simulink model "controller_v9"  (R2022b)
settings: Solver=ode4  StartTime=0.0  StopTime=5  FixedStep=0.00001  RelTol=1e-3
values from neighbouring files (symbols this model uses):
  m = 6    [coordinator_v2.m]
  N = 10    [coordinator_v2.m]
undefined symbols (not defined in the file or in its folder): PD_result, sd, X, Y, Z
libraries: sm_lib x191, nesl_utility x71
(part 2 of 5)

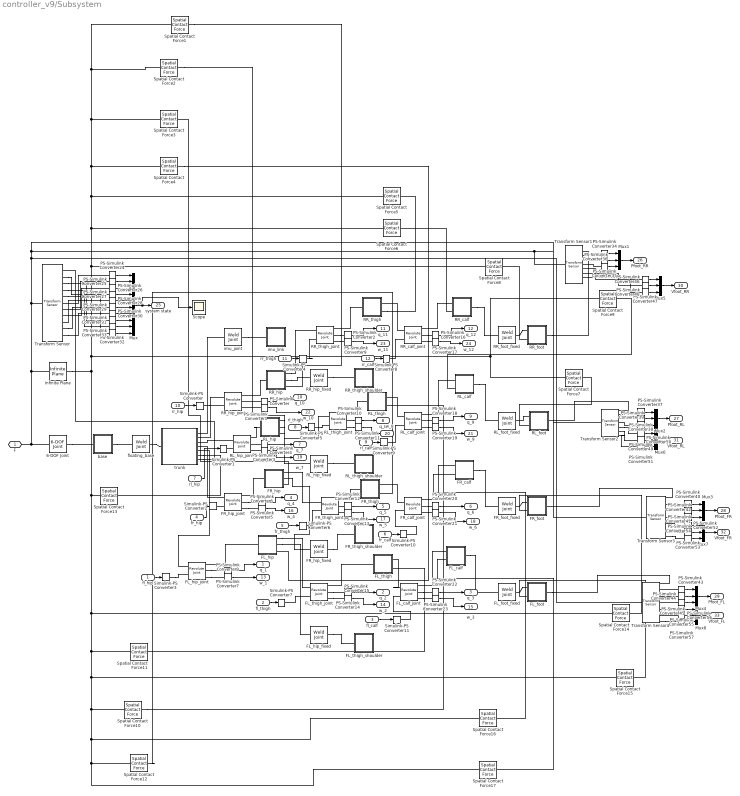
== system controller_v9/Subsystem ==
  fl_hip : Inport
  fl_thigh : Inport  Port=2
  fl_calf : Inport  Port=3
  fr_hip : Inport  Port=4
  fr_thigh : Inport  Port=5
  fr_calf : Inport  Port=6
  rl_hip : Inport  Port=7
  rl_thigh : Inport  Port=8
  rl_calf : Inport  Port=9
  rr_hip : Inport  Port=10
  rr_thigh : Inport  Port=11
  rr_calf : Inport  Port=12
  6-DOF Joint : sm_lib/Joints/6-DOF Joint  JointMode=Normal  SenseConstraintForce=off  SenseConstraintForceX=off  SenseConstraintForceY=off  SenseConstraintForceZ=off  SenseConstraintTorque=off  SenseConstraintTorqueX=off  SenseConstraintTorqueY=off  SenseConstraintTorqueZ=off  SenseTotalForce=off  SenseTotalForceX=off  SenseTotalForceY=off  SenseTotalForceZ=off  SenseTotalTorque=off  SenseTotalTorqueX=off  SenseTotalTorqueY=off  SenseTotalTorqueZ=off  CompositeWrenchDir=FollowerOnBase  CompositeWrenchFrame=BaseFrame  PxEquilibriumPosition=0  PxEquilibriumPositionUnits=m  PxSpringStiffness=0  PxSpringStiffnessUnits=N/m  PxDampingCoefficient=0  PxDampingCoefficientUnits=N/(m/s)  PxTorqueActuationMode=NoTorque  PxMotionActuationMode=ComputedMotion  PxSensePosition=off  PxSenseVelocity=off  PxSenseAcceleration=off  PxSenseTorqueForce=off  PxSenseLowerLimitTorqueForce=off  PxSenseUpperLimitTorqueForce=off  PxLowerLimitSpecify=off  PxLowerLimitBound=-1  PxLowerLimitBoundUnits=m  PxLowerLimitStiffness=1e6  PxLowerLimitStiffnessUnits=N/m  PxLowerLimitDamping=1e3  PxLowerLimitDampingUnits=N/(m/s)  PxLowerLimitTransitionRegionWidth=1e-4  PxLowerLimitTransitionRegionWidthUnits=m  PxUpperLimitSpecify=off  PxUpperLimitBound=1  PxUpperLimitBoundUnits=m  PxUpperLimitStiffness=1e6  PxUpperLimitStiffnessUnits=N/m  PxUpperLimitDamping=1e3  PxUpperLimitDampingUnits=N/(m/s)  PxUpperLimitTransitionRegionWidth=1e-4  PxUpperLimitTransitionRegionWidthUnits=m  PxPositionTargetSpecify=off  PxPositionTargetPriority=High  PxPositionTargetValue=0  PxPositionTargetValueUnits=m  PxVelocityTargetSpecify=off  PxVelocityTargetPriority=High  PxVelocityTargetValue=0  PxVelocityTargetValueUnits=m/s  PyEquilibriumPosition=0  PyEquilibriumPositionUnits=m  PySpringStiffness=0  PySpringStiffnessUnits=N/m  PyDampingCoefficient=0  PyDampingCoefficientUnits=N/(m/s)  PyTorqueActuationMode=NoTorque  PyMotionActuationMode=ComputedMotion  PySensePosition=off  PySenseVelocity=off  PySenseAcceleration=off  PySenseTorqueForce=off  PySenseLowerLimitTorqueForce=off  PySenseUpperLimitTorqueForce=off  PyLowerLimitSpecify=off  PyLowerLimitBound=-1  PyLowerLimitBoundUnits=m  PyLowerLimitStiffness=1e6  PyLowerLimitStiffnessUnits=N/m  PyLowerLimitDamping=1e3  PyLowerLimitDampingUnits=N/(m/s)  PyLowerLimitTransitionRegionWidth=1e-4  PyLowerLimitTransitionRegionWidthUnits=m  PyUpperLimitSpecify=off  PyUpperLimitBound=1  PyUpperLimitBoundUnits=m  PyUpperLimitStiffness=1e6  PyUpperLimitStiffnessUnits=N/m  PyUpperLimitDamping=1e3  PyUpperLimitDampingUnits=N/(m/s)  PyUpperLimitTransitionRegionWidth=1e-4  PyUpperLimitTransitionRegionWidthUnits=m  PyPositionTargetSpecify=off  PyPositionTargetPriority=High  PyPositionTargetValue=0  PyPositionTargetValueUnits=m  PyVelocityTargetSpecify=off  PyVelocityTargetPriority=High  PyVelocityTargetValue=0  PyVelocityTargetValueUnits=m/s  PzEquilibriumPosition=0  PzEquilibriumPositionUnits=m  PzSpringStiffness=0  PzSpringStiffnessUnits=N/m  PzDampingCoefficient=0  PzDampingCoefficientUnits=N/(m/s)  PzTorqueActuationMode=NoTorque  PzMotionActuationMode=ComputedMotion  PzSensePosition=off  PzSenseVelocity=off  PzSenseAcceleration=off  PzSenseTorqueForce=off  PzSenseLowerLimitTorqueForce=off  PzSenseUpperLimitTorqueForce=off  PzLowerLimitSpecify=off  PzLowerLimitBound=-1  PzLowerLimitBoundUnits=m  PzLowerLimitStiffness=1e6  PzLowerLimitStiffnessUnits=N/m  PzLowerLimitDamping=1e3  PzLowerLimitDampingUnits=N/(m/s)  PzLowerLimitTransitionRegionWidth=1e-4  PzLowerLimitTransitionRegionWidthUnits=m  PzUpperLimitSpecify=off  PzUpperLimitBound=1  PzUpperLimitBoundUnits=m  PzUpperLimitStiffness=1e6  PzUpperLimitStiffnessUnits=N/m  PzUpperLimitDamping=1e3  PzUpperLimitDampingUnits=N/(m/s)  PzUpperLimitTransitionRegionWidth=1e-4  PzUpperLimitTransitionRegionWidthUnits=m  PzPositionTargetSpecify=on  PzPositionTargetPriority=High  PzPositionTargetValue=0.3  PzPositionTargetValueUnits=m  PzVelocityTargetSpecify=off  PzVelocityTargetPriority=High  PzVelocityTargetValue=0  PzVelocityTargetValueUnits=m/s  SphEqPosRotationMethod=None  SphEqPosRotationAngleUnits=deg  SphEqPosRotationStandardAxis=+Z  SphEqPosRotationAngle=0.0  SphEqPosRotationArbitraryAxis=[0 0 1]  SphEqPosFollAlignAxisA=+X  SphEqPosBaseAlignAxisA=+Y  SphEqPosFollAlignAxisB=+Y  SphEqPosBaseAlignAxisB=+Z  SphEqPosRotationSequenceAxes=FollowerAxes  SphEqPosRotationSequence=XYX  SphEqPosRotationSequenceAngles=[0 0 0]  SphEqPosRotationSequenceAnglesUnits=deg  SphEqPosRotationMatrix=[1 0 0; 0 1 0; 0 0 1]  SphEqPosQuaternion=[1 0 0 0]  SphSpringStiffness=0  SphSpringStiffnessUnits=N*m/deg  SphDampingCoefficient=0  SphDampingCoefficientUnits=N*m/(deg/s)  SphActuateTorqueX=off  SphActuateTorqueY=off  SphActuateTorqueZ=off  SphActuateTorque=off  SphTorqueActuationMode=NoTorque  SphMotionActuationMode=ComputedMotion  SphActuationFrame=BaseFrame  SphSensePosition=off  SphSenseVelocityX=off  SphSenseVelocityY=off  SphSenseVelocityZ=off  SphSenseVelocity=off  SphSenseAccelerationX=off  SphSenseAccelerationY=off  SphSenseAccelerationZ=off  SphSenseAcceleration=off  SphSenseTorqueX=off  SphSenseTorqueY=off  SphSenseTorqueZ=off  SphSenseTorqueForce=off  SphSenseLowerLimitTorqueMag=off  SphSenseUpperLimitTorqueMag=off  SphSensingFrame=BaseFrame  SphLowerLimitSpecify=off  SphLowerLimitBound=15  SphLowerLimitBoundUnits=deg  SphLowerLimitStiffness=1e4  SphLowerLimitStiffnessUnits=N*m/deg  SphLowerLimitDamping=10  SphLowerLimitDampingUnits=N*m/(deg/s)  SphLowerLimitTransitionRegionWidth=0.1  SphLowerLimitTransitionRegionWidthUnits=deg  SphUpperLimitSpecify=off  SphUpperLimitBound=45  SphUpperLimitBoundUnits=deg  SphUpperLimitStiffness=1e4  SphUpperLimitStiffnessUnits=N*m/deg  SphUpperLimitDamping=10  SphUpperLimitDampingUnits=N*m/(deg/s)  SphUpperLimitTransitionRegionWidth=0.1  SphUpperLimitTransitionRegionWidthUnits=deg  SphPositionTargetRotationMethod=None  SphPositionTargetRotationAngleUnits=deg  SphPositionTargetRotationStandardAxis=+Z  SphPositionTargetRotationAngle=0.0  SphPositionTargetRotationArbitraryAxis=[0 0 1]  SphPositionTargetFollAlignAxisA=+X  SphPositionTargetBaseAlignAxisA=+Y  SphPositionTargetFollAlignAxisB=+Y  SphPositionTargetBaseAlignAxisB=+Z  SphPositionTargetRotationSequenceAxes=FollowerAxes  SphPositionTargetRotationSequence=XYX  SphPositionTargetRotationSequenceAngles=[0 0 0]  SphPositionTargetRotationSequenceAnglesUnits=deg  SphPositionTargetRotationMatrix=[1 0 0; 0 1 0; 0 0 1]  SphPositionTargetQuaternion=[1 0 0 0]  SphPositionTargetSpecify=off  SphPositionTargetPriority=High  SphVelocityTargetValue=[0 0 0]  SphVelocityTargetValueUnits=deg/s  SphVelocityTargetSpecify=off  SphVelocityTargetPriority=High  SphVelocityTargetInFollowerFrame=on
  FL_calf : Subsystem
  FL_calf_joint : sm_lib/Joints/Revolute Joint  JointMode=Normal  SenseConstraintForce=off  SenseConstraintForceX=off  SenseConstraintForceY=off  SenseConstraintForceZ=off  SenseConstraintTorque=off  SenseConstraintTorqueX=off  SenseConstraintTorqueY=off  SenseConstraintTorqueZ=off  SenseTotalForce=off  SenseTotalForceX=off  SenseTotalForceY=off  SenseTotalForceZ=off  SenseTotalTorque=off  SenseTotalTorqueX=off  SenseTotalTorqueY=off  SenseTotalTorqueZ=off  CompositeWrenchDir=FollowerOnBase  CompositeWrenchFrame=BaseFrame  EquilibriumPosition=0  EquilibriumPositionUnits=deg  SpringStiffness=0  SpringStiffnessUnits=N*m/deg  DampingCoefficient=0.01  DampingCoefficientUnits=kg*m^2/(rad*s)  TorqueActuationMode=InputTorque  MotionActuationMode=ComputedMotion  SensePosition=on  SenseVelocity=on  SenseAcceleration=off  SenseTorqueForce=off  SenseLowerLimitTorqueForce=off  SenseUpperLimitTorqueForce=off  LowerLimitSpecify=on  LowerLimitBound=-2.69653369433  LowerLimitBoundUnits=rad  LowerLimitStiffness=1e4  LowerLimitStiffnessUnits=N*m/deg  LowerLimitDamping=10  LowerLimitDampingUnits=N*m/(deg/s)  LowerLimitTransitionRegionWidth=0.1  LowerLimitTransitionRegionWidthUnits=deg  UpperLimitSpecify=on  UpperLimitBound=-0.916297857297  UpperLimitBoundUnits=rad  UpperLimitStiffness=1e4  UpperLimitStiffnessUnits=N*m/deg  UpperLimitDamping=10  UpperLimitDampingUnits=N*m/(deg/s)  UpperLimitTransitionRegionWidth=0.1  UpperLimitTransitionRegionWidthUnits=deg  PositionTargetSpecify=on  PositionTargetPriority=High  PositionTargetValue=-90  PositionTargetValueUnits=deg  VelocityTargetSpecify=off  VelocityTargetPriority=High  VelocityTargetValue=0  VelocityTargetValueUnits=deg/s
  FL_foot : Subsystem
  FL_foot_fixed : sm_lib/Joints/Weld Joint  JointMode=Normal  SenseConstraintForce=off  SenseConstraintForceX=off  SenseConstraintForceY=off  SenseConstraintForceZ=off  SenseConstraintTorque=off  SenseConstraintTorqueX=off  SenseConstraintTorqueY=off  SenseConstraintTorqueZ=off  SenseTotalForce=off  SenseTotalForceX=off  SenseTotalForceY=off  SenseTotalForceZ=off  SenseTotalTorque=off  SenseTotalTorqueX=off  SenseTotalTorqueY=off  SenseTotalTorqueZ=off  CompositeWrenchDir=FollowerOnBase  CompositeWrenchFrame=BaseFrame
  FL_hip : Subsystem
  FL_hip_fixed : sm_lib/Joints/Weld Joint  JointMode=Normal  SenseConstraintForce=off  SenseConstraintForceX=off  SenseConstraintForceY=off  SenseConstraintForceZ=off  SenseConstraintTorque=off  SenseConstraintTorqueX=off  SenseConstraintTorqueY=off  SenseConstraintTorqueZ=off  SenseTotalForce=off  SenseTotalForceX=off  SenseTotalForceY=off  SenseTotalForceZ=off  SenseTotalTorque=off  SenseTotalTorqueX=off  SenseTotalTorqueY=off  SenseTotalTorqueZ=off  CompositeWrenchDir=FollowerOnBase  CompositeWrenchFrame=BaseFrame
  FL_hip_joint : sm_lib/Joints/Revolute Joint  JointMode=Normal  SenseConstraintForce=off  SenseConstraintForceX=off  SenseConstraintForceY=off  SenseConstraintForceZ=off  SenseConstraintTorque=off  SenseConstraintTorqueX=off  SenseConstraintTorqueY=off  SenseConstraintTorqueZ=off  SenseTotalForce=off  SenseTotalForceX=off  SenseTotalForceY=off  SenseTotalForceZ=off  SenseTotalTorque=off  SenseTotalTorqueX=off  SenseTotalTorqueY=off  SenseTotalTorqueZ=off  CompositeWrenchDir=FollowerOnBase  CompositeWrenchFrame=BaseFrame  EquilibriumPosition=0  EquilibriumPositionUnits=deg  SpringStiffness=0  SpringStiffnessUnits=N*m/deg  DampingCoefficient=0.01  DampingCoefficientUnits=kg*m^2/(rad*s)  TorqueActuationMode=InputTorque  MotionActuationMode=ComputedMotion  SensePosition=on  SenseVelocity=on  SenseAcceleration=off  SenseTorqueForce=off  SenseLowerLimitTorqueForce=off  SenseUpperLimitTorqueForce=off  LowerLimitSpecify=on  LowerLimitBound=-0.802851455917  LowerLimitBoundUnits=rad  LowerLimitStiffness=1e4  LowerLimitStiffnessUnits=N*m/deg  LowerLimitDamping=10  LowerLimitDampingUnits=N*m/(deg/s)  LowerLimitTransitionRegionWidth=0.1  LowerLimitTransitionRegionWidthUnits=deg  UpperLimitSpecify=on  UpperLimitBound=0.802851455917  UpperLimitBoundUnits=rad  UpperLimitStiffness=1e4  UpperLimitStiffnessUnits=N*m/deg  UpperLimitDamping=10  UpperLimitDampingUnits=N*m/(deg/s)  UpperLimitTransitionRegionWidth=0.1  UpperLimitTransitionRegionWidthUnits=deg  PositionTargetSpecify=off  PositionTargetPriority=High  PositionTargetValue=0  PositionTargetValueUnits=deg  VelocityTargetSpecify=off  VelocityTargetPriority=High  VelocityTargetValue=0  VelocityTargetValueUnits=deg/s
  FL_thigh : Subsystem
  FL_thigh_joint : sm_lib/Joints/Revolute Joint  JointMode=Normal  SenseConstraintForce=off  SenseConstraintForceX=off  SenseConstraintForceY=off  SenseConstraintForceZ=off  SenseConstraintTorque=off  SenseConstraintTorqueX=off  SenseConstraintTorqueY=off  SenseConstraintTorqueZ=off  SenseTotalForce=off  SenseTotalForceX=off  SenseTotalForceY=off  SenseTotalForceZ=off  SenseTotalTorque=off  SenseTotalTorqueX=off  SenseTotalTorqueY=off  SenseTotalTorqueZ=off  CompositeWrenchDir=FollowerOnBase  CompositeWrenchFrame=BaseFrame  EquilibriumPosition=0  EquilibriumPositionUnits=deg  SpringStiffness=0  SpringStiffnessUnits=N*m/deg  DampingCoefficient=0.01  DampingCoefficientUnits=kg*m^2/(rad*s)  TorqueActuationMode=InputTorque  MotionActuationMode=ComputedMotion  SensePosition=on  SenseVelocity=on  SenseAcceleration=off  SenseTorqueForce=off  SenseLowerLimitTorqueForce=off  SenseUpperLimitTorqueForce=off  LowerLimitSpecify=on  LowerLimitBound=-1.0471975512  LowerLimitBoundUnits=rad  LowerLimitStiffness=1e4  LowerLimitStiffnessUnits=N*m/deg  LowerLimitDamping=10  LowerLimitDampingUnits=N*m/(deg/s)  LowerLimitTransitionRegionWidth=0.1  LowerLimitTransitionRegionWidthUnits=deg  UpperLimitSpecify=on  UpperLimitBound=4.18879020479  UpperLimitBoundUnits=rad  UpperLimitStiffness=1e4  UpperLimitStiffnessUnits=N*m/deg  UpperLimitDamping=10  UpperLimitDampingUnits=N*m/(deg/s)  UpperLimitTransitionRegionWidth=0.1  UpperLimitTransitionRegionWidthUnits=deg  PositionTargetSpecify=on  PositionTargetPriority=High  PositionTargetValue=15  PositionTargetValueUnits=deg  VelocityTargetSpecify=off  VelocityTargetPriority=High  VelocityTargetValue=0  VelocityTargetValueUnits=deg/s
  FL_thigh_shoulder : Subsystem
  FR_calf : Subsystem
  FR_calf_joint : sm_lib/Joints/Revolute Joint  JointMode=Normal  SenseConstraintForce=off  SenseConstraintForceX=off  SenseConstraintForceY=off  SenseConstraintForceZ=off  SenseConstraintTorque=off  SenseConstraintTorqueX=off  SenseConstraintTorqueY=off  SenseConstraintTorqueZ=off  SenseTotalForce=off  SenseTotalForceX=off  SenseTotalForceY=off  SenseTotalForceZ=off  SenseTotalTorque=off  SenseTotalTorqueX=off  SenseTotalTorqueY=off  SenseTotalTorqueZ=off  CompositeWrenchDir=FollowerOnBase  CompositeWrenchFrame=BaseFrame  EquilibriumPosition=0  EquilibriumPositionUnits=deg  SpringStiffness=0  SpringStiffnessUnits=N*m/deg  DampingCoefficient=0.01  DampingCoefficientUnits=kg*m^2/(rad*s)  TorqueActuationMode=InputTorque  MotionActuationMode=ComputedMotion  SensePosition=on  SenseVelocity=on  SenseAcceleration=off  SenseTorqueForce=off  SenseLowerLimitTorqueForce=off  SenseUpperLimitTorqueForce=off  LowerLimitSpecify=on  LowerLimitBound=-2.69653369433  LowerLimitBoundUnits=rad  LowerLimitStiffness=1e4  LowerLimitStiffnessUnits=N*m/deg  LowerLimitDamping=10  LowerLimitDampingUnits=N*m/(deg/s)  LowerLimitTransitionRegionWidth=0.1  LowerLimitTransitionRegionWidthUnits=deg  UpperLimitSpecify=on  UpperLimitBound=-0.916297857297  UpperLimitBoundUnits=rad  UpperLimitStiffness=1e4  UpperLimitStiffnessUnits=N*m/deg  UpperLimitDamping=10  UpperLimitDampingUnits=N*m/(deg/s)  UpperLimitTransitionRegionWidth=0.1  UpperLimitTransitionRegionWidthUnits=deg  PositionTargetSpecify=on  PositionTargetPriority=High  PositionTargetValue=-90  PositionTargetValueUnits=deg  VelocityTargetSpecify=off  VelocityTargetPriority=High  VelocityTargetValue=0  VelocityTargetValueUnits=deg/s
  FR_foot : Subsystem
  FR_foot_fixed : sm_lib/Joints/Weld Joint  JointMode=Normal  SenseConstraintForce=off  SenseConstraintForceX=off  SenseConstraintForceY=off  SenseConstraintForceZ=off  SenseConstraintTorque=off  SenseConstraintTorqueX=off  SenseConstraintTorqueY=off  SenseConstraintTorqueZ=off  SenseTotalForce=off  SenseTotalForceX=off  SenseTotalForceY=off  SenseTotalForceZ=off  SenseTotalTorque=off  SenseTotalTorqueX=off  SenseTotalTorqueY=off  SenseTotalTorqueZ=off  CompositeWrenchDir=FollowerOnBase  CompositeWrenchFrame=BaseFrame
  FR_hip : Subsystem
  FR_hip_fixed : sm_lib/Joints/Weld Joint  JointMode=Normal  SenseConstraintForce=off  SenseConstraintForceX=off  SenseConstraintForceY=off  SenseConstraintForceZ=off  SenseConstraintTorque=off  SenseConstraintTorqueX=off  SenseConstraintTorqueY=off  SenseConstraintTorqueZ=off  SenseTotalForce=off  SenseTotalForceX=off  SenseTotalForceY=off  SenseTotalForceZ=off  SenseTotalTorque=off  SenseTotalTorqueX=off  SenseTotalTorqueY=off  SenseTotalTorqueZ=off  CompositeWrenchDir=FollowerOnBase  CompositeWrenchFrame=BaseFrame
  FR_hip_joint : sm_lib/Joints/Revolute Joint  JointMode=Normal  SenseConstraintForce=off  SenseConstraintForceX=off  SenseConstraintForceY=off  SenseConstraintForceZ=off  SenseConstraintTorque=off  SenseConstraintTorqueX=off  SenseConstraintTorqueY=off  SenseConstraintTorqueZ=off  SenseTotalForce=off  SenseTotalForceX=off  SenseTotalForceY=off  SenseTotalForceZ=off  SenseTotalTorque=off  SenseTotalTorqueX=off  SenseTotalTorqueY=off  SenseTotalTorqueZ=off  CompositeWrenchDir=FollowerOnBase  CompositeWrenchFrame=BaseFrame  EquilibriumPosition=0  EquilibriumPositionUnits=deg  SpringStiffness=0  SpringStiffnessUnits=N*m/deg  DampingCoefficient=0.01  DampingCoefficientUnits=kg*m^2/(rad*s)  TorqueActuationMode=InputTorque  MotionActuationMode=ComputedMotion  SensePosition=on  SenseVelocity=on  SenseAcceleration=off  SenseTorqueForce=off  SenseLowerLimitTorqueForce=off  SenseUpperLimitTorqueForce=off  LowerLimitSpecify=on  LowerLimitBound=-0.802851455917  LowerLimitBoundUnits=rad  LowerLimitStiffness=1e4  LowerLimitStiffnessUnits=N*m/deg  LowerLimitDamping=10  LowerLimitDampingUnits=N*m/(deg/s)  LowerLimitTransitionRegionWidth=0.1  LowerLimitTransitionRegionWidthUnits=deg  UpperLimitSpecify=on  UpperLimitBound=0.802851455917  UpperLimitBoundUnits=rad  UpperLimitStiffness=1e4  UpperLimitStiffnessUnits=N*m/deg  UpperLimitDamping=10  UpperLimitDampingUnits=N*m/(deg/s)  UpperLimitTransitionRegionWidth=0.1  UpperLimitTransitionRegionWidthUnits=deg  PositionTargetSpecify=off  PositionTargetPriority=High  PositionTargetValue=0  PositionTargetValueUnits=deg  VelocityTargetSpecify=off  VelocityTargetPriority=High  VelocityTargetValue=0  VelocityTargetValueUnits=deg/s
  FR_thigh : Subsystem
  FR_thigh_joint : sm_lib/Joints/Revolute Joint  JointMode=Normal  SenseConstraintForce=off  SenseConstraintForceX=off  SenseConstraintForceY=off  SenseConstraintForceZ=off  SenseConstraintTorque=off  SenseConstraintTorqueX=off  SenseConstraintTorqueY=off  SenseConstraintTorqueZ=off  SenseTotalForce=off  SenseTotalForceX=off  SenseTotalForceY=off  SenseTotalForceZ=off  SenseTotalTorque=off  SenseTotalTorqueX=off  SenseTotalTorqueY=off  SenseTotalTorqueZ=off  CompositeWrenchDir=FollowerOnBase  CompositeWrenchFrame=BaseFrame  EquilibriumPosition=0  EquilibriumPositionUnits=deg  SpringStiffness=0  SpringStiffnessUnits=N*m/deg  DampingCoefficient=0.01  DampingCoefficientUnits=kg*m^2/(rad*s)  TorqueActuationMode=InputTorque  MotionActuationMode=ComputedMotion  SensePosition=on  SenseVelocity=on  SenseAcceleration=off  SenseTorqueForce=off  SenseLowerLimitTorqueForce=off  SenseUpperLimitTorqueForce=off  LowerLimitSpecify=on  LowerLimitBound=-1.0471975512  LowerLimitBoundUnits=rad  LowerLimitStiffness=1e4  LowerLimitStiffnessUnits=N*m/deg  LowerLimitDamping=10  LowerLimitDampingUnits=N*m/(deg/s)  LowerLimitTransitionRegionWidth=0.1  LowerLimitTransitionRegionWidthUnits=deg  UpperLimitSpecify=on  UpperLimitBound=4.18879020479  UpperLimitBoundUnits=rad  UpperLimitStiffness=1e4  UpperLimitStiffnessUnits=N*m/deg  UpperLimitDamping=10  UpperLimitDampingUnits=N*m/(deg/s)  UpperLimitTransitionRegionWidth=0.1  UpperLimitTransitionRegionWidthUnits=deg  PositionTargetSpecify=on  PositionTargetPriority=High  PositionTargetValue=15  PositionTargetValueUnits=deg  VelocityTargetSpecify=off  VelocityTargetPriority=High  VelocityTargetValue=0  VelocityTargetValueUnits=deg/s
  FR_thigh_shoulder : Subsystem
  Infinite Plane : sm_lib/Curves and Surfaces/Infinite Plane  GraphicType=Rectangle  GraphicPlaneWidth=10  GraphicPlaneWidthUnits=m  GraphicPlaneHeight=10  GraphicPlaneHeightUnits=m  GraphicVisPropType=SimpleVisualProperties  GraphicDiffuseColor=[0.5 0.5 0.5]  GraphicOpacity=0.25  GraphicSpecularColor=[0.5 0.5 0.5 1.0]  GraphicAmbientColor=[0.15 0.15 0.15 1.0]  GraphicEmissiveColor=[0.0 0.0 0.0 1.0]  GraphicShininess=75
  Mux : Mux  Inputs=10
  Mux{1..8} (8 alike) : Mux  Inputs=3
  PS-Simulink Converter{,1..57} (58 alike) : nesl_utility/PS-Simulink Converter  PhysicalDomain=network_engine_domain  SubClassName=ps_output  LeftPortType=input  RightPortType=output  PseudoPeriodic=off  Frequencies=[]  VectorFormat=inherit  Unit=inherit  AffineConversion=off
  RL_calf : Subsystem
  RL_calf_joint : sm_lib/Joints/Revolute Joint  JointMode=Normal  SenseConstraintForce=off  SenseConstraintForceX=off  SenseConstraintForceY=off  SenseConstraintForceZ=off  SenseConstraintTorque=off  SenseConstraintTorqueX=off  SenseConstraintTorqueY=off  SenseConstraintTorqueZ=off  SenseTotalForce=off  SenseTotalForceX=off  SenseTotalForceY=off  SenseTotalForceZ=off  SenseTotalTorque=off  SenseTotalTorqueX=off  SenseTotalTorqueY=off  SenseTotalTorqueZ=off  CompositeWrenchDir=FollowerOnBase  CompositeWrenchFrame=BaseFrame  EquilibriumPosition=0  EquilibriumPositionUnits=deg  SpringStiffness=0  SpringStiffnessUnits=N*m/deg  DampingCoefficient=0.01  DampingCoefficientUnits=kg*m^2/(rad*s)  TorqueActuationMode=InputTorque  MotionActuationMode=ComputedMotion  SensePosition=on  SenseVelocity=on  SenseAcceleration=off  SenseTorqueForce=off  SenseLowerLimitTorqueForce=off  SenseUpperLimitTorqueForce=off  LowerLimitSpecify=on  LowerLimitBound=-2.69653369433  LowerLimitBoundUnits=rad  LowerLimitStiffness=1e4  LowerLimitStiffnessUnits=N*m/deg  LowerLimitDamping=10  LowerLimitDampingUnits=N*m/(deg/s)  LowerLimitTransitionRegionWidth=0.1  LowerLimitTransitionRegionWidthUnits=deg  UpperLimitSpecify=on  UpperLimitBound=-0.916297857297  UpperLimitBoundUnits=rad  UpperLimitStiffness=1e4  UpperLimitStiffnessUnits=N*m/deg  UpperLimitDamping=10  UpperLimitDampingUnits=N*m/(deg/s)  UpperLimitTransitionRegionWidth=0.1  UpperLimitTransitionRegionWidthUnits=deg  PositionTargetSpecify=on  PositionTargetPriority=High  PositionTargetValue=-90  PositionTargetValueUnits=deg  VelocityTargetSpecify=off  VelocityTargetPriority=High  VelocityTargetValue=0  VelocityTargetValueUnits=deg/s
  RL_foot : Subsystem
  RL_foot_fixed : sm_lib/Joints/Weld Joint  JointMode=Normal  SenseConstraintForce=off  SenseConstraintForceX=off  SenseConstraintForceY=off  SenseConstraintForceZ=off  SenseConstraintTorque=off  SenseConstraintTorqueX=off  SenseConstraintTorqueY=off  SenseConstraintTorqueZ=off  SenseTotalForce=off  SenseTotalForceX=off  SenseTotalForceY=off  SenseTotalForceZ=off  SenseTotalTorque=off  SenseTotalTorqueX=off  SenseTotalTorqueY=off  SenseTotalTorqueZ=off  CompositeWrenchDir=FollowerOnBase  CompositeWrenchFrame=BaseFrame
  RL_hip : Subsystem
  RL_hip_fixed : sm_lib/Joints/Weld Joint  JointMode=Normal  SenseConstraintForce=off  SenseConstraintForceX=off  SenseConstraintForceY=off  SenseConstraintForceZ=off  SenseConstraintTorque=off  SenseConstraintTorqueX=off  SenseConstraintTorqueY=off  SenseConstraintTorqueZ=off  SenseTotalForce=off  SenseTotalForceX=off  SenseTotalForceY=off  SenseTotalForceZ=off  SenseTotalTorque=off  SenseTotalTorqueX=off  SenseTotalTorqueY=off  SenseTotalTorqueZ=off  CompositeWrenchDir=FollowerOnBase  CompositeWrenchFrame=BaseFrame
  RL_hip_joint : sm_lib/Joints/Revolute Joint  JointMode=Normal  SenseConstraintForce=off  SenseConstraintForceX=off  SenseConstraintForceY=off  SenseConstraintForceZ=off  SenseConstraintTorque=off  SenseConstraintTorqueX=off  SenseConstraintTorqueY=off  SenseConstraintTorqueZ=off  SenseTotalForce=off  SenseTotalForceX=off  SenseTotalForceY=off  SenseTotalForceZ=off  SenseTotalTorque=off  SenseTotalTorqueX=off  SenseTotalTorqueY=off  SenseTotalTorqueZ=off  CompositeWrenchDir=FollowerOnBase  CompositeWrenchFrame=BaseFrame  EquilibriumPosition=0  EquilibriumPositionUnits=deg  SpringStiffness=0  SpringStiffnessUnits=N*m/deg  DampingCoefficient=0.01  DampingCoefficientUnits=kg*m^2/(rad*s)  TorqueActuationMode=InputTorque  MotionActuationMode=ComputedMotion  SensePosition=on  SenseVelocity=on  SenseAcceleration=off  SenseTorqueForce=off  SenseLowerLimitTorqueForce=off  SenseUpperLimitTorqueForce=off  LowerLimitSpecify=on  LowerLimitBound=-0.802851455917  LowerLimitBoundUnits=rad  LowerLimitStiffness=1e4  LowerLimitStiffnessUnits=N*m/deg  LowerLimitDamping=10  LowerLimitDampingUnits=N*m/(deg/s)  LowerLimitTransitionRegionWidth=0.1  LowerLimitTransitionRegionWidthUnits=deg  UpperLimitSpecify=on  UpperLimitBound=0.802851455917  UpperLimitBoundUnits=rad  UpperLimitStiffness=1e4  UpperLimitStiffnessUnits=N*m/deg  UpperLimitDamping=10  UpperLimitDampingUnits=N*m/(deg/s)  UpperLimitTransitionRegionWidth=0.1  UpperLimitTransitionRegionWidthUnits=deg  PositionTargetSpecify=off  PositionTargetPriority=High  PositionTargetValue=0  PositionTargetValueUnits=deg  VelocityTargetSpecify=off  VelocityTargetPriority=High  VelocityTargetValue=0  VelocityTargetValueUnits=deg/s
  RL_thigh : Subsystem
  RL_thigh_joint : sm_lib/Joints/Revolute Joint  JointMode=Normal  SenseConstraintForce=off  SenseConstraintForceX=off  SenseConstraintForceY=off  SenseConstraintForceZ=off  SenseConstraintTorque=off  SenseConstraintTorqueX=off  SenseConstraintTorqueY=off  SenseConstraintTorqueZ=off  SenseTotalForce=off  SenseTotalForceX=off  SenseTotalForceY=off  SenseTotalForceZ=off  SenseTotalTorque=off  SenseTotalTorqueX=off  SenseTotalTorqueY=off  SenseTotalTorqueZ=off  CompositeWrenchDir=FollowerOnBase  CompositeWrenchFrame=BaseFrame  EquilibriumPosition=0  EquilibriumPositionUnits=deg  SpringStiffness=0  SpringStiffnessUnits=N*m/deg  DampingCoefficient=0.01  DampingCoefficientUnits=kg*m^2/(rad*s)  TorqueActuationMode=InputTorque  MotionActuationMode=ComputedMotion  SensePosition=on  SenseVelocity=on  SenseAcceleration=off  SenseTorqueForce=off  SenseLowerLimitTorqueForce=off  SenseUpperLimitTorqueForce=off  LowerLimitSpecify=on  LowerLimitBound=-1.0471975512  LowerLimitBoundUnits=rad  LowerLimitStiffness=1e4  LowerLimitStiffnessUnits=N*m/deg  LowerLimitDamping=10  LowerLimitDampingUnits=N*m/(deg/s)  LowerLimitTransitionRegionWidth=0.1  LowerLimitTransitionRegionWidthUnits=deg  UpperLimitSpecify=on  UpperLimitBound=4.18879020479  UpperLimitBoundUnits=rad  UpperLimitStiffness=1e4  UpperLimitStiffnessUnits=N*m/deg  UpperLimitDamping=10  UpperLimitDampingUnits=N*m/(deg/s)  UpperLimitTransitionRegionWidth=0.1  UpperLimitTransitionRegionWidthUnits=deg  PositionTargetSpecify=on  PositionTargetPriority=High  PositionTargetValue=15  PositionTargetValueUnits=deg  VelocityTargetSpecify=off  VelocityTargetPriority=High  VelocityTargetValue=0  VelocityTargetValueUnits=deg/s
  RL_thigh_shoulder : Subsystem
  RR_calf : Subsystem
  RR_calf_joint : sm_lib/Joints/Revolute Joint  JointMode=Normal  SenseConstraintForce=off  SenseConstraintForceX=off  SenseConstraintForceY=off  SenseConstraintForceZ=off  SenseConstraintTorque=off  SenseConstraintTorqueX=off  SenseConstraintTorqueY=off  SenseConstraintTorqueZ=off  SenseTotalForce=off  SenseTotalForceX=off  SenseTotalForceY=off  SenseTotalForceZ=off  SenseTotalTorque=off  SenseTotalTorqueX=off  SenseTotalTorqueY=off  SenseTotalTorqueZ=off  CompositeWrenchDir=FollowerOnBase  CompositeWrenchFrame=BaseFrame  EquilibriumPosition=0  EquilibriumPositionUnits=deg  SpringStiffness=0  SpringStiffnessUnits=N*m/deg  DampingCoefficient=0.01  DampingCoefficientUnits=kg*m^2/(rad*s)  TorqueActuationMode=InputTorque  MotionActuationMode=ComputedMotion  SensePosition=on  SenseVelocity=on  SenseAcceleration=off  SenseTorqueForce=off  SenseLowerLimitTorqueForce=off  SenseUpperLimitTorqueForce=off  LowerLimitSpecify=on  LowerLimitBound=-2.69653369433  LowerLimitBoundUnits=rad  LowerLimitStiffness=1e4  LowerLimitStiffnessUnits=N*m/deg  LowerLimitDamping=10  LowerLimitDampingUnits=N*m/(deg/s)  LowerLimitTransitionRegionWidth=0.1  LowerLimitTransitionRegionWidthUnits=deg  UpperLimitSpecify=on  UpperLimitBound=-0.916297857297  UpperLimitBoundUnits=rad  UpperLimitStiffness=1e4  UpperLimitStiffnessUnits=N*m/deg  UpperLimitDamping=10  UpperLimitDampingUnits=N*m/(deg/s)  UpperLimitTransitionRegionWidth=0.1  UpperLimitTransitionRegionWidthUnits=deg  PositionTargetSpecify=on  PositionTargetPriority=High  PositionTargetValue=-90  PositionTargetValueUnits=deg  VelocityTargetSpecify=off  VelocityTargetPriority=High  VelocityTargetValue=0  VelocityTargetValueUnits=deg/s
  RR_foot : Subsystem
  RR_foot_fixed : sm_lib/Joints/Weld Joint  JointMode=Normal  SenseConstraintForce=off  SenseConstraintForceX=off  SenseConstraintForceY=off  SenseConstraintForceZ=off  SenseConstraintTorque=off  SenseConstraintTorqueX=off  SenseConstraintTorqueY=off  SenseConstraintTorqueZ=off  SenseTotalForce=off  SenseTotalForceX=off  SenseTotalForceY=off  SenseTotalForceZ=off  SenseTotalTorque=off  SenseTotalTorqueX=off  SenseTotalTorqueY=off  SenseTotalTorqueZ=off  CompositeWrenchDir=FollowerOnBase  CompositeWrenchFrame=BaseFrame
  RR_hip : Subsystem
  RR_hip_fixed : sm_lib/Joints/Weld Joint  JointMode=Normal  SenseConstraintForce=off  SenseConstraintForceX=off  SenseConstraintForceY=off  SenseConstraintForceZ=off  SenseConstraintTorque=off  SenseConstraintTorqueX=off  SenseConstraintTorqueY=off  SenseConstraintTorqueZ=off  SenseTotalForce=off  SenseTotalForceX=off  SenseTotalForceY=off  SenseTotalForceZ=off  SenseTotalTorque=off  SenseTotalTorqueX=off  SenseTotalTorqueY=off  SenseTotalTorqueZ=off  CompositeWrenchDir=FollowerOnBase  CompositeWrenchFrame=BaseFrame
  RR_hip_joint : sm_lib/Joints/Revolute Joint  JointMode=Normal  SenseConstraintForce=off  SenseConstraintForceX=off  SenseConstraintForceY=off  SenseConstraintForceZ=off  SenseConstraintTorque=off  SenseConstraintTorqueX=off  SenseConstraintTorqueY=off  SenseConstraintTorqueZ=off  SenseTotalForce=off  SenseTotalForceX=off  SenseTotalForceY=off  SenseTotalForceZ=off  SenseTotalTorque=off  SenseTotalTorqueX=off  SenseTotalTorqueY=off  SenseTotalTorqueZ=off  CompositeWrenchDir=FollowerOnBase  CompositeWrenchFrame=BaseFrame  EquilibriumPosition=0  EquilibriumPositionUnits=deg  SpringStiffness=0  SpringStiffnessUnits=N*m/deg  DampingCoefficient=0.01  DampingCoefficientUnits=kg*m^2/(rad*s)  TorqueActuationMode=InputTorque  MotionActuationMode=ComputedMotion  SensePosition=on  SenseVelocity=on  SenseAcceleration=off  SenseTorqueForce=off  SenseLowerLimitTorqueForce=off  SenseUpperLimitTorqueForce=off  LowerLimitSpecify=on  LowerLimitBound=-0.802851455917  LowerLimitBoundUnits=rad  LowerLimitStiffness=1e4  LowerLimitStiffnessUnits=N*m/deg  LowerLimitDamping=10  LowerLimitDampingUnits=N*m/(deg/s)  LowerLimitTransitionRegionWidth=0.1  LowerLimitTransitionRegionWidthUnits=deg  UpperLimitSpecify=on  UpperLimitBound=0.802851455917  UpperLimitBoundUnits=rad  UpperLimitStiffness=1e4  UpperLimitStiffnessUnits=N*m/deg  UpperLimitDamping=10  UpperLimitDampingUnits=N*m/(deg/s)  UpperLimitTransitionRegionWidth=0.1  UpperLimitTransitionRegionWidthUnits=deg  PositionTargetSpecify=off  PositionTargetPriority=High  PositionTargetValue=0  PositionTargetValueUnits=deg  VelocityTargetSpecify=off  VelocityTargetPriority=High  VelocityTargetValue=0  VelocityTargetValueUnits=deg/s
  RR_thigh : Subsystem
  RR_thigh_joint : sm_lib/Joints/Revolute Joint  JointMode=Normal  SenseConstraintForce=off  SenseConstraintForceX=off  SenseConstraintForceY=off  SenseConstraintForceZ=off  SenseConstraintTorque=off  SenseConstraintTorqueX=off  SenseConstraintTorqueY=off  SenseConstraintTorqueZ=off  SenseTotalForce=off  SenseTotalForceX=off  SenseTotalForceY=off  SenseTotalForceZ=off  SenseTotalTorque=off  SenseTotalTorqueX=off  SenseTotalTorqueY=off  SenseTotalTorqueZ=off  CompositeWrenchDir=FollowerOnBase  CompositeWrenchFrame=BaseFrame  EquilibriumPosition=0  EquilibriumPositionUnits=deg  SpringStiffness=0  SpringStiffnessUnits=N*m/deg  DampingCoefficient=0.01  DampingCoefficientUnits=kg*m^2/(rad*s)  TorqueActuationMode=InputTorque  MotionActuationMode=ComputedMotion  SensePosition=on  SenseVelocity=on  SenseAcceleration=off  SenseTorqueForce=off  SenseLowerLimitTorqueForce=off  SenseUpperLimitTorqueForce=off  LowerLimitSpecify=on  LowerLimitBound=-1.0471975512  LowerLimitBoundUnits=rad  LowerLimitStiffness=1e4  LowerLimitStiffnessUnits=N*m/deg  LowerLimitDamping=10  LowerLimitDampingUnits=N*m/(deg/s)  LowerLimitTransitionRegionWidth=0.1  LowerLimitTransitionRegionWidthUnits=deg  UpperLimitSpecify=on  UpperLimitBound=4.18879020479  UpperLimitBoundUnits=rad  UpperLimitStiffness=1e4  UpperLimitStiffnessUnits=N*m/deg  UpperLimitDamping=10  UpperLimitDampingUnits=N*m/(deg/s)  UpperLimitTransitionRegionWidth=0.1  UpperLimitTransitionRegionWidthUnits=deg  PositionTargetSpecify=on  PositionTargetPriority=High  PositionTargetValue=15  PositionTargetValueUnits=deg  VelocityTargetSpecify=off  VelocityTargetPriority=High  VelocityTargetValue=0  VelocityTargetValueUnits=deg/s
  RR_thigh_shoulder : Subsystem
  Scope : Scope
  Simulink-PS Converter{,1..11} (12 alike) : nesl_utility/Simulink-PS Converter  PhysicalDomain=network_engine_domain  SubClassName=ps_input  LeftPortType=input  RightPortType=output  PseudoPeriodic=off  Frequencies=[]  NoiseDistribution=none  NoiseParameters=[]  Unit=1  AffineConversion=off  FilteringAndDerivatives=provide  SimscapeFilterOrder=1  InputFilterTimeConstant=0.001  UdotUserProvided=0
  Spatial Contact Force{1..17} (17 alike) : sm_lib/Forces and Torques/Spatial Contact Force  SenseContactBaseRotation=off  SenseContactBaseTranslation=off  CoefficientOfDynamicFriction=100  CoefficientOfStaticFriction=100  NormalDamping=1e3  NormalDampingUnits=N/(m/s)  SenseContactSignal=off  NormalStiffness=1e6  NormalStiffnessUnits=N/m  FrictionalCriticalVelocity=1e-3  FrictionalCriticalVelocityUnits=m/s  ZeroCrossDetectContactStartAndEnd=off  SenseContactFollowerRotation=off  SenseContactFollowerTranslation=off  FrictionType=SmoothStickSlip  SenseFrictionalForceMagnitude=off  SenseNormalForceMagnitude=off  NormalForceType=SmoothSpringDamper  SenseNormalVelocity=off  SenseSeparationDistance=off  SenseTangentialVelocity=off  NormalTransitionRegionWidth=1e-4  NormalTransitionRegionWidthUnits=m
  Transform Sensor : sm_lib/Frames and Transforms/Transform Sensor  MeasurementFrame=World  SenseAngle=off  SenseAxis=off  SenseQ=off  SenseR=off  SenseRotationSequence=on  RotationSequence=XYZ  SenseOmegaX=on  SenseOmegaY=on  SenseOmegaZ=on  SenseQDot=off  SenseRDot=off  SenseAlphaX=off  SenseAlphaY=off  SenseAlphaZ=off  SenseQDDot=off  SenseRDDot=off  SenseX=on  SenseY=on  SenseZ=on  SenseRad=off  SenseAzim=off  SenseDist=off  SenseInc=off  SenseXDot=on  SenseYDot=on  SenseZDot=on  SenseRadDot=off  SenseAzimDot=off  SenseDistDot=off  SenseIncDot=off  SenseXDDot=off  SenseYDDot=off  SenseZDDot=off  SenseRadDDot=off  SenseAzimDDot=off  SenseDistDDot=off  SenseIncDDot=off
  Transform Sensor{1..4} (4 alike) : sm_lib/Frames and Transforms/Transform Sensor  MeasurementFrame=World  SenseAngle=off  SenseAxis=off  SenseQ=off  SenseR=off  SenseRotationSequence=off  RotationSequence=XYX  SenseOmegaX=off  SenseOmegaY=off  SenseOmegaZ=off  SenseQDot=off  SenseRDot=off  SenseAlphaX=off  SenseAlphaY=off  SenseAlphaZ=off  SenseQDDot=off  SenseRDDot=off  SenseX=on  SenseY=on  SenseZ=on  SenseRad=off  SenseAzim=off  SenseDist=off  SenseInc=off  SenseXDot=on  SenseYDot=on  SenseZDot=on  SenseRadDot=off  SenseAzimDot=off  SenseDistDot=off  SenseIncDot=off  SenseXDDot=off  SenseYDDot=off  SenseZDDot=off  SenseRadDDot=off  SenseAzimDDot=off  SenseDistDDot=off  SenseIncDDot=off
  base : Subsystem
  floating_base : sm_lib/Joints/Weld Joint  JointMode=Normal  SenseConstraintForce=off  SenseConstraintForceX=off  SenseConstraintForceY=off  SenseConstraintForceZ=off  SenseConstraintTorque=off  SenseConstraintTorqueX=off  SenseConstraintTorqueY=off  SenseConstraintTorqueZ=off  SenseTotalForce=off  SenseTotalForceX=off  SenseTotalForceY=off  SenseTotalForceZ=off  SenseTotalTorque=off  SenseTotalTorqueX=off  SenseTotalTorqueY=off  SenseTotalTorqueZ=off  CompositeWrenchDir=FollowerOnBase  CompositeWrenchFrame=BaseFrame
  imu_joint : sm_lib/Joints/Weld Joint  JointMode=Normal  SenseConstraintForce=off  SenseConstraintForceX=off  SenseConstraintForceY=off  SenseConstraintForceZ=off  SenseConstraintTorque=off  SenseConstraintTorqueX=off  SenseConstraintTorqueY=off  SenseConstraintTorqueZ=off  SenseTotalForce=off  SenseTotalForceX=off  SenseTotalForceY=off  SenseTotalForceZ=off  SenseTotalTorque=off  SenseTotalTorqueX=off  SenseTotalTorqueY=off  SenseTotalTorqueZ=off  CompositeWrenchDir=FollowerOnBase  CompositeWrenchFrame=BaseFrame
  imu_link : Subsystem
  trunk : Subsystem
  F : PMIOPort  Side=Left
  q_1 : Outport
  q_2 : Outport  Port=2
  q_3 : Outport  Port=3
  q_4 : Outport  Port=4
  q_5 : Outport  Port=5
  q_6 : Outport  Port=6
  q_7 : Outport  Port=7
  q_8 : Outport  Port=8
  q_9 : Outport  Port=9
  q_10 : Outport  Port=10
  q_11 : Outport  Port=11
  q_12 : Outport  Port=12
  w_1 : Outport  Port=13
  w_2 : Outport  Port=14
  w_3 : Outport  Port=15
  w_4 : Outport  Port=16
  w_5 : Outport  Port=17
  w_6 : Outport  Port=18
  w_7 : Outport  Port=19
  w_8 : Outport  Port=20
  w_9 : Outport  Port=21
  w_10 : Outport  Port=22
  w_11 : Outport  Port=23
  w_12 : Outport  Port=24
  system state : Outport  Port=25
  Pfoot_RR : Outport  Port=26
  Pfoot_RL : Outport  Port=27
  Pfoot_FR : Outport  Port=28
  Pfoot_FL : Outport  Port=29
  Vfoot_RR : Outport  Port=30
  Vfoot_RL : Outport  Port=31
  Vfoot_FR : Outport  Port=32
  Vfoot_FL : Outport  Port=33
  wires:
  PS-Simulink Converter13/1 -> w_5/1
  PS-Simulink Converter8/1 -> w_1/1
  PS-Simulink Converter/1 -> q_10/1
  PS-Simulink Converter22/1 -> q_3/1
  PS-Simulink Converter4/1 -> w_7/1
  PS-Simulink Converter6/1 -> w_4/1
  PS-Simulink Converter18/1 -> q_9/1
  PS-Simulink Converter7/1 -> q_1/1
  PS-Simulink Converter5/1 -> q_4/1
  PS-Simulink Converter3/1 -> q_7/1
  PS-Simulink Converter1/1 -> w_10/1
  PS-Simulink Converter15/1 -> w_2/1
  PS-Simulink Converter14/1 -> q_2/1
  PS-Simulink Converter2/1 -> q_11/1
  PS-Simulink Converter9/1 -> w_11/1
  PS-Simulink Converter19/1 -> w_9/1
  PS-Simulink Converter11/1 -> w_8/1
  PS-Simulink Converter10/1 -> q_8/1
  PS-Simulink Converter20/1 -> q_6/1
  PS-Simulink Converter16/1 -> q_12/1
  PS-Simulink Converter17/1 -> w_12/1
  PS-Simulink Converter12/1 -> q_5/1
  PS-Simulink Converter23/1 -> w_3/1
  PS-Simulink Converter21/1 -> w_6/1
  rr_hip/1 -> Simulink-PS Converter/1
  rl_hip/1 -> Simulink-PS Converter1/1
  fr_hip/1 -> Simulink-PS Converter2/1
  fl_hip/1 -> Simulink-PS Converter3/1
  rr_thigh/1 -> Simulink-PS Converter4/1
  rl_thigh/1 -> Simulink-PS Converter5/1
  fr_thigh/1 -> Simulink-PS Converter6/1
  fl_thigh/1 -> Simulink-PS Converter7/1
  rr_calf/1 -> Simulink-PS Converter8/1
  rl_calf/1 -> Simulink-PS Converter9/1
  fr_calf/1 -> Simulink-PS Converter10/1
  fl_calf/1 -> Simulink-PS Converter11/1
  PS-Simulink Converter24/1 -> Mux/1
  PS-Simulink Converter25/1 -> Mux/2
  PS-Simulink Converter26/1 -> Mux/3
  PS-Simulink Converter27/1 -> Mux/4
  PS-Simulink Converter28/1 -> Mux/5
  PS-Simulink Converter29/1 -> Mux/6
  PS-Simulink Converter30/1 -> Mux/7
  PS-Simulink Converter31/1 -> Mux/8
  PS-Simulink Converter32/1 -> Mux/9
  PS-Simulink Converter33/1 -> Mux/10
  Mux/1 -> Scope/1, system state/1
  Mux1/1 -> Pfoot_RR/1
  PS-Simulink Converter34/1 -> Mux1/1
  PS-Simulink Converter35/1 -> Mux1/2
  PS-Simulink Converter36/1 -> Mux1/3
  Mux2/1 -> Pfoot_RL/1
  PS-Simulink Converter39/1 -> Mux2/3
  PS-Simulink Converter37/1 -> Mux2/1
  PS-Simulink Converter38/1 -> Mux2/2
  PS-Simulink Converter42/1 -> Mux3/3
  Mux3/1 -> Pfoot_FR/1
  PS-Simulink Converter41/1 -> Mux3/2
  PS-Simulink Converter40/1 -> Mux3/1
  PS-Simulink Converter43/1 -> Mux4/1
  Mux4/1 -> Pfoot_FL/1
  PS-Simulink Converter45/1 -> Mux4/3
  PS-Simulink Converter44/1 -> Mux4/2
  PS-Simulink Converter48/1 -> Mux5/3
  PS-Simulink Converter47/1 -> Mux5/2
  PS-Simulink Converter46/1 -> Mux5/1
  Mux5/1 -> Vfoot_RR/1
  PS-Simulink Converter51/1 -> Mux6/3
  PS-Simulink Converter50/1 -> Mux6/2
  PS-Simulink Converter49/1 -> Mux6/1
  Mux6/1 -> Vfoot_RL/1
  PS-Simulink Converter54/1 -> Mux7/3
  PS-Simulink Converter53/1 -> Mux7/2
  PS-Simulink Converter52/1 -> Mux7/1
  Mux7/1 -> Vfoot_FR/1
  PS-Simulink Converter56/1 -> Mux8/2
  PS-Simulink Converter57/1 -> Mux8/3
  Mux8/1 -> Vfoot_FL/1
  PS-Simulink Converter55/1 -> Mux8/1
  connections:
  FR_hip/RConn1 -- FR_thigh_joint/LConn1
  base/RConn1 -- floating_base/LConn1
  FR_calf_joint/RConn3 -- PS-Simulink Converter21/LConn1
  RR_hip_fixed/RConn1 -- RR_thigh_shoulder/LConn1
  RR_calf_joint/LConn1 -- RR_thigh/RConn1
  FL_hip_fixed/RConn1 -- FL_thigh_shoulder/LConn1
  RR_hip_joint/LConn1 -- trunk/RConn2
  FL_thigh_joint/RConn2 -- PS-Simulink Converter14/LConn1
  FL_calf/LConn1 -- FL_calf_joint/RConn1
  RR_calf/RConn1 -- RR_foot_fixed/LConn1
  RL_foot/LConn1 -- RL_foot_fixed/RConn1
  RL_hip/RConn1 -- RL_thigh_joint/LConn1
  FL_thigh/LConn1 -- FL_thigh_joint/RConn1
  FL_hip/RConn2 -- FL_hip_fixed/LConn1
  PS-Simulink Converter4/LConn1 -- RL_hip_joint/RConn3
  FL_hip/RConn1 -- FL_thigh_joint/LConn1
  FL_calf_joint/LConn1 -- FL_thigh/RConn1
  PS-Simulink Converter1/LConn1 -- RR_hip_joint/RConn3
  FL_hip_joint/LConn1 -- trunk/RConn5
  FL_calf_joint/RConn3 -- PS-Simulink Converter23/LConn1
  FR_calf_joint/RConn2 -- PS-Simulink Converter20/LConn1
  imu_joint/RConn1 -- imu_link/LConn1
  RL_calf_joint/LConn1 -- RL_thigh/RConn1
  imu_joint/LConn1 -- trunk/RConn1
  RL_thigh_joint/RConn3 -- PS-Simulink Converter11/LConn1
  FR_foot/LConn1 -- FR_foot_fixed/RConn1
  FR_thigh/LConn1 -- FR_thigh_joint/RConn1
  FR_hip_joint/LConn1 -- trunk/RConn4
  RL_hip_joint/LConn1 -- trunk/RConn3
  RL_hip/LConn1 -- RL_hip_joint/RConn1
  FL_calf_joint/RConn2 -- PS-Simulink Converter22/LConn1
  RL_calf/LConn1 -- RL_calf_joint/RConn1
  RL_hip/RConn2 -- RL_hip_fixed/LConn1
  PS-Simulink Converter/LConn1 -- RR_hip_joint/RConn2
  FL_calf/RConn1 -- FL_foot_fixed/LConn1
  FL_thigh_joint/RConn3 -- PS-Simulink Converter15/LConn1
  floating_base/RConn1 -- trunk/LConn1
  FR_hip/LConn1 -- FR_hip_joint/RConn1
  FR_calf/LConn1 -- FR_calf_joint/RConn1
  FR_hip_fixed/RConn1 -- FR_thigh_shoulder/LConn1
  FR_calf_joint/LConn1 -- FR_thigh/RConn1
  RL_thigh/LConn1 -- RL_thigh_joint/RConn1
  RL_thigh_joint/RConn2 -- PS-Simulink Converter10/LConn1
  RR_thigh/LConn1 -- RR_thigh_joint/RConn1
  RR_calf/LConn1 -- RR_calf_joint/RConn1
  RL_hip_fixed/RConn1 -- RL_thigh_shoulder/LConn1
  RL_calf/RConn1 -- RL_foot_fixed/LConn1
  FR_hip/RConn2 -- FR_hip_fixed/LConn1
  FR_calf/RConn1 -- FR_foot_fixed/LConn1
  FL_foot/LConn1 -- FL_foot_fixed/RConn1
  FL_hip/LConn1 -- FL_hip_joint/RConn1
  FR_thigh_joint/RConn2 -- PS-Simulink Converter12/LConn1
  RR_hip/RConn1 -- RR_thigh_joint/LConn1
  RR_hip/LConn1 -- RR_hip_joint/RConn1
  RR_hip/RConn2 -- RR_hip_fixed/LConn1
  RR_foot/LConn1 -- RR_foot_fixed/RConn1
  FR_thigh_joint/RConn3 -- PS-Simulink Converter13/LConn1
  RR_thigh_joint/RConn2 -- PS-Simulink Converter2/LConn1
  RR_thigh_joint/RConn3 -- PS-Simulink Converter9/LConn1
  PS-Simulink Converter3/LConn1 -- RL_hip_joint/RConn2
  FR_hip_joint/RConn2 -- PS-Simulink Converter5/LConn1
  FR_hip_joint/RConn3 -- PS-Simulink Converter6/LConn1
  FL_hip_joint/RConn3 -- PS-Simulink Converter8/LConn1
  FL_hip_joint/RConn2 -- PS-Simulink Converter7/LConn1
  RL_calf_joint/RConn2 -- PS-Simulink Converter18/LConn1
  RL_calf_joint/RConn3 -- PS-Simulink Converter19/LConn1
  RR_calf_joint/RConn2 -- PS-Simulink Converter16/LConn1
  RR_calf_joint/RConn3 -- PS-Simulink Converter17/LConn1
  Simulink-PS Converter/RConn1 -- RR_hip_joint/LConn2
  Simulink-PS Converter1/RConn1 -- RL_hip_joint/LConn2
  FR_hip_joint/LConn2 -- Simulink-PS Converter2/RConn1
  Simulink-PS Converter3/RConn1 -- FL_hip_joint/LConn2
  Simulink-PS Converter4/RConn1 -- RR_thigh_joint/LConn2
  Simulink-PS Converter5/RConn1 -- RL_thigh_joint/LConn2
  FR_thigh_joint/LConn2 -- Simulink-PS Converter6/RConn1
  FL_thigh_joint/LConn2 -- Simulink-PS Converter7/RConn1
  RR_calf_joint/LConn2 -- Simulink-PS Converter8/RConn1
  RL_calf_joint/LConn2 -- Simulink-PS Converter9/RConn1
  FR_calf_joint/LConn2 -- Simulink-PS Converter10/RConn1
  FL_calf_joint/LConn2 -- Simulink-PS Converter11/RConn1
  6-DOF Joint/RConn1 -- base/LConn1
  6-DOF Joint/LConn1 -- Transform Sensor2/LConn1 -- Transform Sensor3/LConn1 -- Transform Sensor1/LConn1 -- Transform Sensor4/LConn1 -- Transform Sensor/LConn1 -- Infinite Plane/LConn1 -- F/RConn1
  Infinite Plane/RConn1 -- Spatial Contact Force13/LConn1 -- Spatial Contact Force16/LConn1 -- Spatial Contact Force17/LConn1 -- Spatial Contact Force12/LConn1 -- Spatial Contact Force10/LConn1 -- Spatial Contact Force15/LConn1 -- Spatial Contact Force11/LConn1 -- Spatial Contact Force14/LConn1 -- Spatial Contact Force8/LConn1 -- Spatial Contact Force6/LConn1 -- Spatial Contact Force5/LConn1 -- Spatial Contact Force1/LConn1 -- Spatial Contact Force2/LConn1 -- Spatial Contact Force3/LConn1 -- Spatial Contact Force4/LConn1 -- Spatial Contact Force9/LConn1 -- Spatial Contact Force7/LConn1
  Spatial Contact Force1/RConn1 -- RR_hip/RConn3
  Spatial Contact Force2/RConn1 -- RL_hip/RConn3
  FR_hip/RConn3 -- Spatial Contact Force3/RConn1
  Spatial Contact Force4/RConn1 -- FL_hip/RConn3
  RR_thigh/RConn2 -- Spatial Contact Force5/RConn1
  RR_calf/LConn2 -- Spatial Contact Force6/RConn1
  RR_foot/LConn2 -- Spatial Contact Force8/RConn1
  RL_foot/LConn2 -- Spatial Contact Force7/RConn1
  RL_calf/LConn2 -- Spatial Contact Force9/RConn1
  FL_thigh/RConn2 -- Spatial Contact Force11/RConn1
  Spatial Contact Force10/RConn1 -- RL_thigh/RConn2
  FR_foot/LConn2 -- Spatial Contact Force14/RConn1
  FL_foot/LConn2 -- Spatial Contact Force15/RConn1
  FR_calf/LConn2 -- Spatial Contact Force16/RConn1
  FL_calf/LConn2 -- Spatial Contact Force17/RConn1
  Spatial Contact Force12/RConn1 -- FR_thigh/RConn2
  trunk/RConn6 -- Spatial Contact Force13/RConn1
  trunk/RConn7 -- Transform Sensor/RConn1
  Transform Sensor/RConn6 -- PS-Simulink Converter24/LConn1
  Transform Sensor/RConn7 -- PS-Simulink Converter25/LConn1
  Transform Sensor/RConn8 -- PS-Simulink Converter26/LConn1
  Transform Sensor/RConn2 -- PS-Simulink Converter27/LConn1
  Transform Sensor/RConn9 -- PS-Simulink Converter28/LConn1
  Transform Sensor/RConn10 -- PS-Simulink Converter29/LConn1
  Transform Sensor/RConn11 -- PS-Simulink Converter30/LConn1
  Transform Sensor/RConn3 -- PS-Simulink Converter31/LConn1
  Transform Sensor/RConn4 -- PS-Simulink Converter32/LConn1
  Transform Sensor/RConn5 -- PS-Simulink Converter33/LConn1
  RR_foot/RConn1 -- Transform Sensor1/RConn1
  PS-Simulink Converter34/LConn1 -- Transform Sensor1/RConn2
  PS-Simulink Converter35/LConn1 -- Transform Sensor1/RConn3
  PS-Simulink Converter36/LConn1 -- Transform Sensor1/RConn4
  PS-Simulink Converter37/LConn1 -- Transform Sensor2/RConn2
  PS-Simulink Converter38/LConn1 -- Transform Sensor2/RConn3
  PS-Simulink Converter39/LConn1 -- Transform Sensor2/RConn4
  Transform Sensor2/RConn1 -- RL_foot/RConn1
  PS-Simulink Converter41/LConn1 -- Transform Sensor3/RConn3
  PS-Simulink Converter42/LConn1 -- Transform Sensor3/RConn4
  PS-Simulink Converter40/LConn1 -- Transform Sensor3/RConn2
  Transform Sensor3/RConn1 -- FR_foot/RConn1
  PS-Simulink Converter43/LConn1 -- Transform Sensor4/RConn2
  FL_foot/RConn1 -- Transform Sensor4/RConn1
  PS-Simulink Converter44/LConn1 -- Transform Sensor4/RConn3
  PS-Simulink Converter45/LConn1 -- Transform Sensor4/RConn4
  PS-Simulink Converter46/LConn1 -- Transform Sensor1/RConn5
  PS-Simulink Converter47/LConn1 -- Transform Sensor1/RConn6
  PS-Simulink Converter48/LConn1 -- Transform Sensor1/RConn7
  Transform Sensor2/RConn5 -- PS-Simulink Converter49/LConn1
  Transform Sensor2/RConn6 -- PS-Simulink Converter50/LConn1
  Transform Sensor2/RConn7 -- PS-Simulink Converter51/LConn1
  Transform Sensor3/RConn5 -- PS-Simulink Converter52/LConn1
  Transform Sensor3/RConn6 -- PS-Simulink Converter53/LConn1
  Transform Sensor3/RConn7 -- PS-Simulink Converter54/LConn1
  Transform Sensor4/RConn5 -- PS-Simulink Converter55/LConn1
  Transform Sensor4/RConn6 -- PS-Simulink Converter56/LConn1
  Transform Sensor4/RConn7 -- PS-Simulink Converter57/LConn1
